simulink model "APP_System_Rev_0"  (R2022b)
settings: Solver=VariableStepAuto  StartTime=0.0  StopTime=1  MaxStep=1e-3  RelTol=1e-3
libraries: simulink x1
settings Model: Creator=HiTech  LastModifiedBy=HiTech

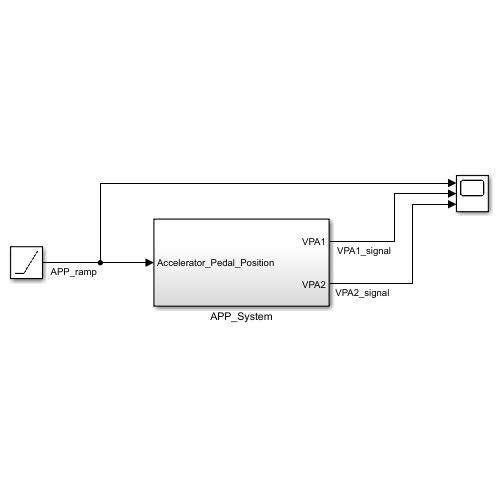
[thumbnail: Simulink's stored preview of the top-level diagram]
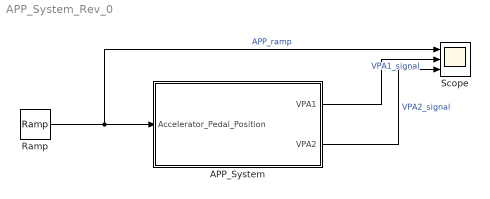
== system APP_System_Rev_0 ==
  APP_System : Subsystem
  Ramp : simulink/Sources/Ramp  slope=1  start=0  InitialOutput=0
  Scope : Scope  NumInputPorts=3
  wires:
  Ramp/1 -> Scope/1, APP_System/1(Accelerator_Pedal_Position)  "APP_ramp"
  APP_System/1(VPA1) -> Scope/2  "VPA1_signal"
  APP_System/2(VPA2) -> Scope/3  "VPA2_signal"

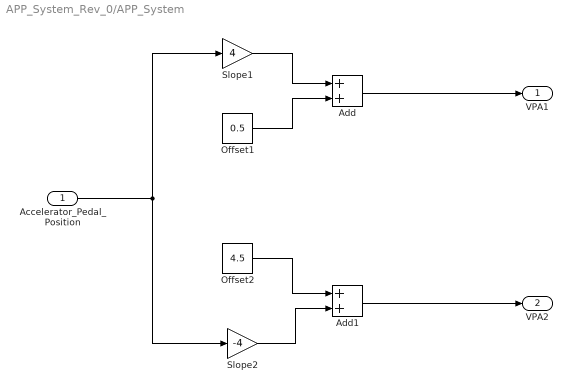
== system APP_System_Rev_0/APP_System ==
  Accelerator_Pedal_Position : Inport
  Add : Sum
  Add1 : Sum
  Offset1 : Constant  Value=0.5
  Offset2 : Constant  Value=4.5
  Slope1 : Gain  Gain=4
  Slope2 : Gain  Gain=-4
  VPA1 : Outport
  VPA2 : Outport  Port=2
  wires:
  Accelerator_Pedal_Position/1 -> Slope1/1, Slope2/1
  Offset2/1 -> Add1/1
  Add/1 -> VPA1/1
  Slope1/1 -> Add/1
  Slope2/1 -> Add1/2
  Offset1/1 -> Add/2
  Add1/1 -> VPA2/1
